simulink model "NonLinearSimulation"  (R2018b)
settings: Solver=VariableStepAuto  StartTime=0.0  StopTime=10.0  RelTol=1e-3
settings Model: Creator=AndyA  LastModifiedBy=AndyA

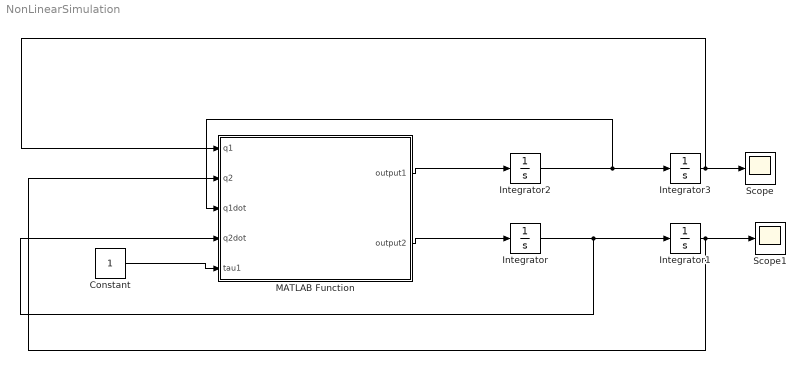
== system NonLinearSimulation ==
  Constant : Constant
  Integrator{,1..3} (4 alike) : Integrator
  MATLAB Function : MATLAB Function  TreatAsAtomicUnit=on
  Scope : Scope
  Scope1 : Scope
  wires:
  Constant/1 -> MATLAB Function/5(tau1)
  MATLAB Function/1(output1) -> Integrator2/1
  Integrator2/1 -> MATLAB Function/3(q1dot), Integrator3/1
  Integrator3/1 -> MATLAB Function/1(q1), Scope/1
  MATLAB Function/2(output2) -> Integrator/1
  Integrator/1 -> MATLAB Function/4(q2dot), Integrator1/1
  Integrator1/1 -> MATLAB Function/2(q2), Scope1/1

== matlab function NonLinearSimulation/MATLAB Function ==
  data: q1 input; output1 output; q2 input; q1dot input; q2dot input; output2 output; tau1 input
function [output1, output2]= NonLinearSimulation(q1, q2 ,q1dot, q2dot,tau1)
output1 = -(tau1 - (3*q1dot)/1000 - (147*cos(q1 + q2))/12500 - (441*cos(q1))/12500 + (3*q2dot^2*sin(q1))/31250 + (15625*((3*cos(q2))/31250 + 32/625)*((3*sin(q1)*q1dot^2)/31250 + (3*q2dot)/5000 + (147*cos(q1 + q2))/12500))/782 + (3*q1dot*q2dot*sin(q1))/15625)/(((3*cos(q2))/15625 + 1567/15625)*((15625*((3*cos(q2))/31250 + 32/625)^2)/(782*((3*cos(q2))/15625 + 1567/15625)) - 1));
output2 = -(tau1 - (3*q1dot)/1000 - (147*cos(q1 + q2))/12500 - (441*cos(q1))/12500 + (3*q2dot^2*sin(q1))/31250 + (3*q1dot*q2dot*sin(q1))/15625 + (((3*cos(q2))/15625 + 1567/15625)*((3*sin(q1)*q1dot^2)/31250 + (3*q2dot)/5000 + (147*cos(q1 + q2))/12500))/((3*cos(q2))/31250 + 32/625))/(((782*((3*cos(q2))/15625 + 1567/15625))/(15625*((3*cos(q2))/31250 + 32/625)^2) - 1)*((3*cos(q2))/31250 + 32/625));
